simulink model "V4_Event_ind_eso_auxi"  (R2021b)
settings: Solver=ode5  StartTime=0.0  StopTime=60.0  FixedStep=0.008  RelTol=1e-3
settings Model: Creator=a1752760  LastModifiedBy=MikeYang

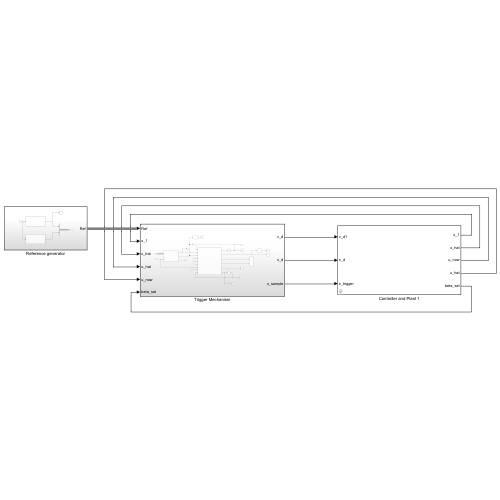
[thumbnail: Simulink's stored preview of the top-level diagram]
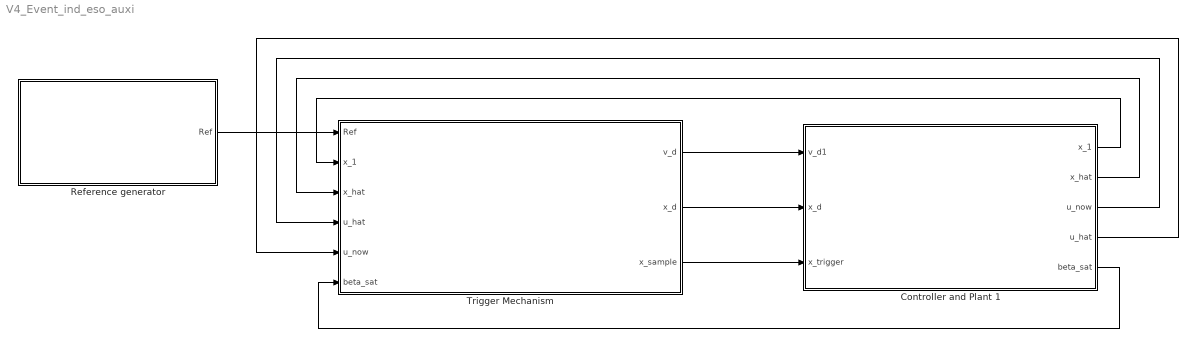
== system V4_Event_ind_eso_auxi ==
  Controller and Plant 1 : Subsystem  mask{InitialCondition=[0.8;-1.1;pi/50], UpperLimit=0.2, LowerLimit=-0.2}
      mask prompts: InitialCondition "Simulink:blkprm_prompts:IntegratorInitCond"; UpperLimit "Simulink:blkprm_prompts:SaturateUpLim"; LowerLimit "Simulink:blkprm_prompts:SaturateLowLim"
      mask TypeOptions InitialCondition: x_int/InitialCondition
      mask TypeOptions UpperLimit: Saturation/UpperLimit
      mask TypeOptions LowerLimit: Saturation/LowerLimit
      mask DialogControl InitialCondition Prompt: 初始条件:
      mask DialogControl UpperLimit Prompt: 上限:
      mask DialogControl LowerLimit Prompt: 下限:
  Reference generator : Subsystem
  Trigger Mechanism : Subsystem
  wires:
  Reference generator/1(Ref) -> Trigger Mechanism/1(Ref)
  Trigger Mechanism/1(v_d) -> Controller and Plant 1/1(v_d1)
  Trigger Mechanism/2(x_d) -> Controller and Plant 1/2(x_d)
  Controller and Plant 1/1(x_1) -> Trigger Mechanism/2(x_1)
  Trigger Mechanism/3(x_sample) -> Controller and Plant 1/3(x_trigger)
  Controller and Plant 1/2(x_hat) -> Trigger Mechanism/3(x_hat)
  Controller and Plant 1/3(u_now) -> Trigger Mechanism/4(u_hat)
  Controller and Plant 1/4(u_hat) -> Trigger Mechanism/5(u_now)
  Controller and Plant 1/5(beta_sat) -> Trigger Mechanism/6(beta_sat)

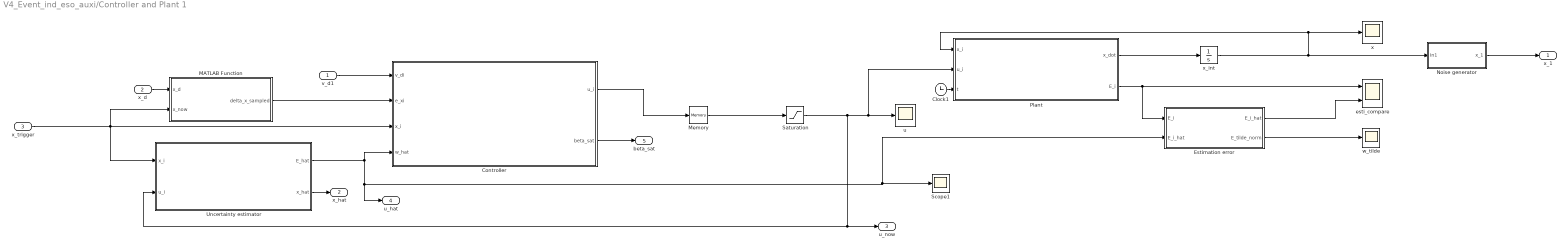
== system V4_Event_ind_eso_auxi/Controller and Plant 1 ==
  v_d1 : Inport
  x_d : Inport  Port=2
  x_trigger : Inport  Port=3
  Clock1 : Clock
  Controller : Subsystem
  Estimation error : MATLAB Function  TreatAsAtomicUnit=on
  MATLAB Function : MATLAB Function  TreatAsAtomicUnit=on
  Memory : Memory  InitialCondition=[0;0;0]
  Noise generator : Subsystem
  Plant : MATLAB Function  TreatAsAtomicUnit=on
  Saturation : Saturate  UpperLimit=UpperLimit  LowerLimit=LowerLimit
  Scope1 : Scope
  Uncertainty estimator : Subsystem  mask{x_hat_1=[0.8;-1.1;pi/50]}
      mask prompts: x_hat_1 "Simulink:blkprm_prompts:IntegratorInitCond"
      mask TypeOptions x_hat_1: Integrator/InitialCondition
      mask DialogControl x_hat_1 Prompt: 初始条件:
  esti_compare : Scope  NumInputPorts=2
  u : Scope
  w_tilde : Scope
  x : Scope
  x_int : Integrator  InitialCondition=InitialCondition
  x_1 : Outport
  x_hat : Outport  Port=2
  u_now : Outport  Port=3
  u_hat : Outport  Port=4
  beta_sat : Outport  Port=5
  wires:
  Plant/2(E_i) -> esti_compare/1, Estimation error/1(E_i)
  Uncertainty estimator/1(E_hat) -> Controller/4(w_hat), u_hat/1, Estimation error/2("E_i_hat "), Scope1/1
  Clock1/1 -> Plant/3(t)
  Plant/1(x_dot) -> x_int/1
  Memory/1 -> Saturation/1
  x_int/1 -> Noise generator/1(In1), Plant/1(x_i), x/1
  v_d1/1 -> Controller/1(v_di)
  Controller/1(u_i) -> Memory/1
  Saturation/1 -> u_now/1, Uncertainty estimator/2(u_i), Plant/2(u_i), u/1
  Estimation error/2(E_tilde_norm) -> w_tilde/1
  Estimation error/1(E_i_hat) -> esti_compare/2
  MATLAB Function/1(delta_x_sampled) -> Controller/2(e_xi)
  x_trigger/1 -> Uncertainty estimator/1(x_i), MATLAB Function/2(x_now), Controller/3(x_i)
  x_d/1 -> MATLAB Function/1(x_d)
  Uncertainty estimator/2(x_hat) -> x_hat/1
  Noise generator/1(x_1) -> x_1/1
  Controller/2(beta_sat) -> beta_sat/1

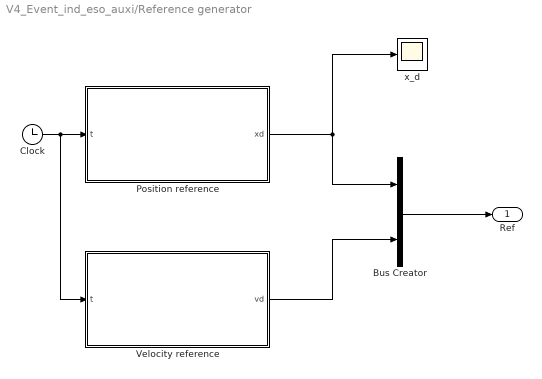
== system V4_Event_ind_eso_auxi/Reference generator ==
  Bus Creator : BusCreator  Inputs=2
  Clock : Clock
  Position reference : MATLAB Function  TreatAsAtomicUnit=on
  Velocity reference : MATLAB Function  TreatAsAtomicUnit=on
  x_d : Scope
  Ref : Outport
  wires:
  Clock/1 -> Velocity reference/1(t), Position reference/1(t)
  Position reference/1(xd) -> x_d/1, Bus Creator/1
  Velocity reference/1(vd) -> Bus Creator/2
  Bus Creator/1 -> Ref/1

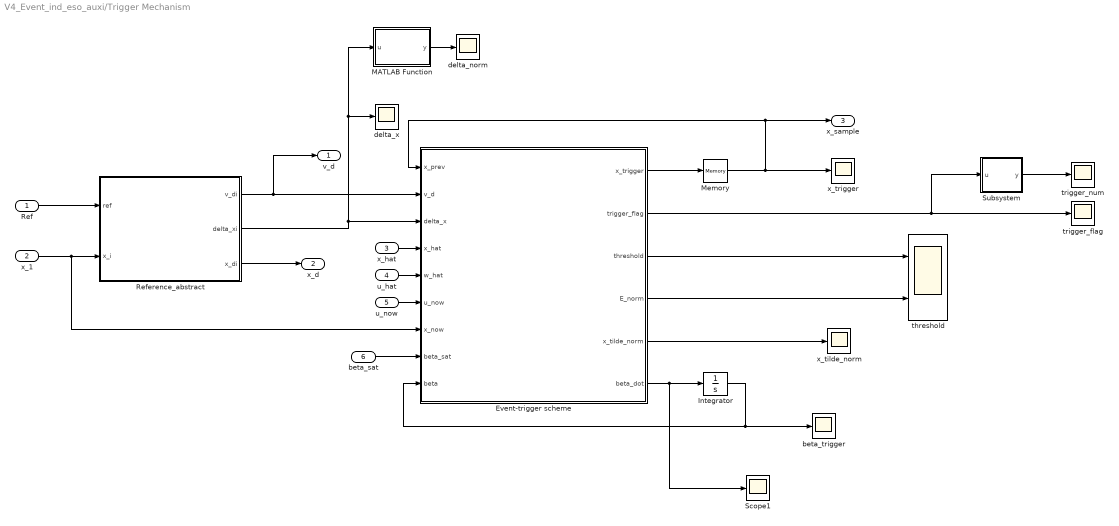
== system V4_Event_ind_eso_auxi/Trigger Mechanism ==
  Ref : Inport
  x_1 : Inport  Port=2
  x_hat : Inport  Port=3
  u_hat : Inport  Port=4
  u_now : Inport  Port=5
  beta_sat : Inport  Port=6
  Event-trigger scheme : MATLAB Function  TreatAsAtomicUnit=on
  Integrator : Integrator  InitialCondition=[2;2]
  MATLAB Function : MATLAB Function  TreatAsAtomicUnit=on
  Memory : Memory  InitialCondition=[0.8;-1.1;pi/50]
  Reference_abstract : MATLAB Function  TreatAsAtomicUnit=on
  Scope1 : Scope
  Subsystem : Subsystem
  beta_trigger : Scope
  delta_norm : Scope
  delta_x : Scope
  threshold : Scope  NumInputPorts=2
  trigger_flag : Scope
  trigger_num : Scope
  x_tilde_norm : Scope
  x_trigger : Scope
  v_d : Outport
  x_d : Outport  Port=2
  x_sample : Outport  Port=3
  wires:
  Ref/1 -> Reference_abstract/1(ref)
  Reference_abstract/1(v_di) -> Event-trigger scheme/2(v_d), v_d/1
  x_1/1 -> Event-trigger scheme/7(x_now), Reference_abstract/2(x_i)
  Event-trigger scheme/1(x_trigger) -> Memory/1
  Memory/1 -> x_trigger/1, x_sample/1, Event-trigger scheme/1(x_prev)
  Reference_abstract/2(delta_xi) -> MATLAB Function/1(u), delta_x/1, Event-trigger scheme/3(delta_x)
  Reference_abstract/3(x_di) -> x_d/1
  x_hat/1 -> Event-trigger scheme/4(x_hat)
  u_hat/1 -> Event-trigger scheme/5(w_hat)
  u_now/1 -> Event-trigger scheme/6(u_now)
  Event-trigger scheme/3(threshold) -> threshold/1
  Event-trigger scheme/4(E_norm) -> threshold/2
  Subsystem/1(y) -> trigger_num/1
  Event-trigger scheme/2(trigger_flag) -> Subsystem/1(u), trigger_flag/1
  Event-trigger scheme/5(x_tilde_norm) -> x_tilde_norm/1
  MATLAB Function/1(y) -> delta_norm/1
  Event-trigger scheme/6(beta_dot) -> Integrator/1, Scope1/1
  Integrator/1 -> beta_trigger/1, Event-trigger scheme/9(beta)
  beta_sat/1 -> Event-trigger scheme/8(beta_sat)

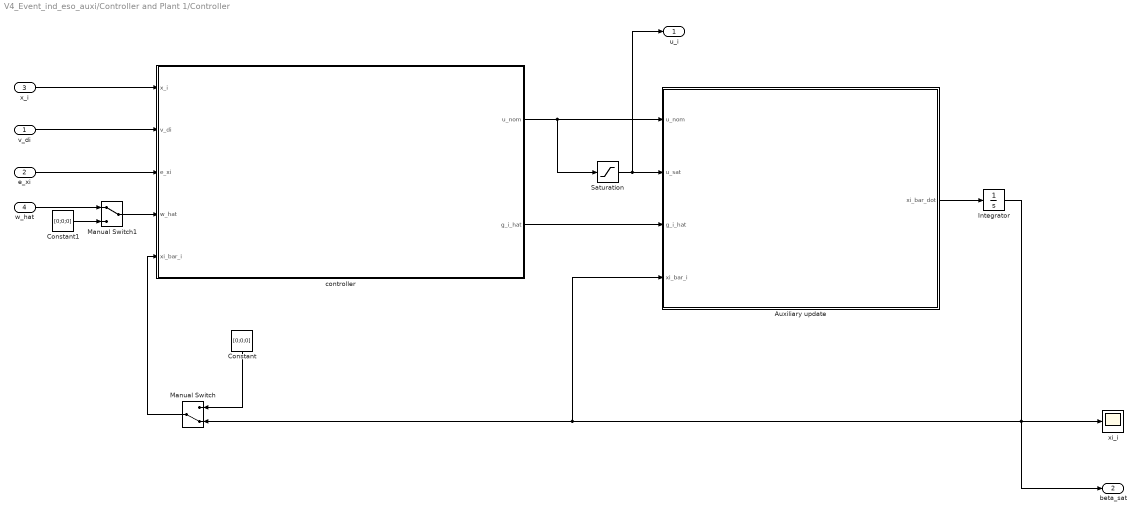
== system V4_Event_ind_eso_auxi/Controller and Plant 1/Controller ==
  v_di : Inport
  e_xi : Inport  Port=2
  x_i : Inport  Port=3
  w_hat : Inport  Port=4
  Auxiliary update : MATLAB Function  TreatAsAtomicUnit=on
  Constant : Constant  Value=[0;0;0]
  Constant1 : Constant  Value=[0;0;0]  VectorParams1D=off
  Integrator : Integrator  InitialCondition=[0.1;0.1;0.1]
  Manual Switch : ManualSwitch  CurrentSetting=0
  Manual Switch1 : ManualSwitch
  Saturation : Saturate  UpperLimit=0.2  LowerLimit=-0.2
  controller : MATLAB Function  TreatAsAtomicUnit=on
  xi_i : Scope
  u_i : Outport
  beta_sat : Outport  Port=2
  wires:
  x_i/1 -> controller/1(x_i)
  v_di/1 -> controller/2(v_di)
  e_xi/1 -> controller/3(e_xi)
  controller/1(u_nom) -> Saturation/1, Auxiliary update/1(u_nom)
  Saturation/1 -> u_i/1, Auxiliary update/2(u_sat)
  controller/2(g_i_hat) -> Auxiliary update/3(g_i_hat)
  Auxiliary update/1(xi_bar_dot) -> Integrator/1
  Constant/1 -> Manual Switch/1
  Manual Switch/1 -> controller/5(xi_bar_i)
  Integrator/1 -> beta_sat/1, xi_i/1, Auxiliary update/4(xi_bar_i), Manual Switch/2
  Constant1/1 -> Manual Switch1/2
  Manual Switch1/1 -> controller/4(w_hat)
  w_hat/1 -> Manual Switch1/1

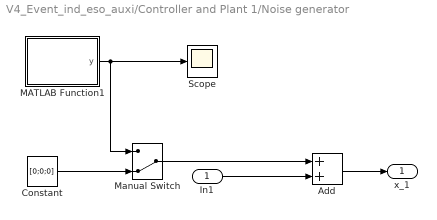
== system V4_Event_ind_eso_auxi/Controller and Plant 1/Noise generator ==
  In1 : Inport
  Add : Sum
  Constant : Constant  Value=[0;0;0]
  MATLAB Function1 : MATLAB Function  TreatAsAtomicUnit=on
  Manual Switch : ManualSwitch  CurrentSetting=0
  Scope : Scope
  x_1 : Outport
  wires:
  MATLAB Function1/1(y) -> Manual Switch/1, Scope/1
  In1/1 -> Add/2
  Add/1 -> x_1/1
  Manual Switch/1 -> Add/1
  Constant/1 -> Manual Switch/2

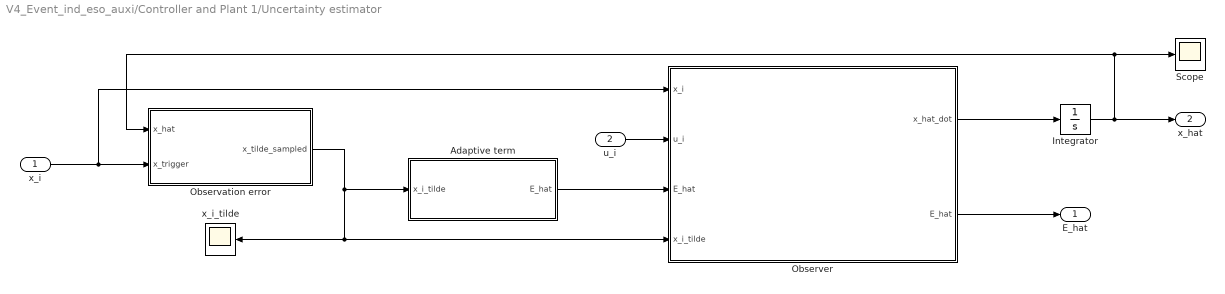
== system V4_Event_ind_eso_auxi/Controller and Plant 1/Uncertainty estimator ==
  x_i : Inport
  u_i : Inport  Port=2
  Adaptive term : Subsystem
  Integrator : Integrator  InitialCondition=x_hat_1
  Observation error : MATLAB Function  TreatAsAtomicUnit=on
  Observer : MATLAB Function  TreatAsAtomicUnit=on
  Scope : Scope
  x_i_tilde : Scope
  E_hat : Outport
  x_hat : Outport  Port=2
  wires:
  Adaptive term/1(E_hat) -> Observer/3("E_hat ")
  Observer/1(x_hat_dot) -> Integrator/1
  u_i/1 -> Observer/2(u_i)
  Integrator/1 -> Observation error/1(x_hat), Scope/1, x_hat/1
  x_i/1 -> Observation error/2(x_trigger), Observer/1(x_i)
  Observer/2(E_hat) -> E_hat/1
  Observation error/1(x_tilde_sampled) -> Observer/4(x_i_tilde), x_i_tilde/1, Adaptive term/1(x_i_tilde)

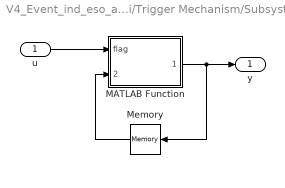
== system V4_Event_ind_eso_auxi/Trigger Mechanism/Subsystem ==
  u : Inport
  MATLAB Function : MATLAB Function  TreatAsAtomicUnit=on
  Memory : Memory
  y : Outport
  wires:
  u/1 -> MATLAB Function/1(flag)
  MATLAB Function/1(number) -> Memory/1, y/1
  Memory/1 -> MATLAB Function/2("number ")

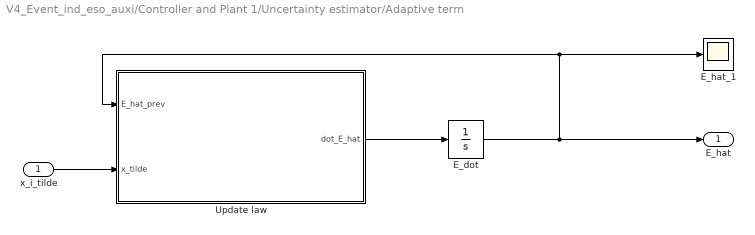
== system V4_Event_ind_eso_auxi/Controller and Plant 1/Uncertainty estimator/Adaptive term ==
  x_i_tilde : Inport
  E_dot : Integrator  InitialCondition=[0;0;0]
  E_hat_1 : Scope
  Update law : MATLAB Function  TreatAsAtomicUnit=on
  E_hat : Outport
  wires:
  E_dot/1 -> Update law/1(E_hat_prev), E_hat_1/1, E_hat/1
  x_i_tilde/1 -> Update law/2(x_tilde)
  Update law/1(dot_E_hat) -> E_dot/1

== matlab function V4_Event_ind_eso_auxi/Trigger Mechanism/Event-trigger scheme ==
  data: x_prev input; v_d input; x_trigger output; delta_x input; x_hat input; w_hat input; u_now input; x_now input; beta_sat input; trigger_flag output; threshold output; E_norm output; x_tilde_norm output; beta input; beta_dot output
function [x_trigger, trigger_flag, threshold, E_norm, x_tilde_norm, beta_dot] = event_trigger(x_prev, v_d, delta_x, x_hat, w_hat, u_now, x_now, beta_sat, beta)

% Observer
eta_1 = [21,21,3];
k_1 = [3,3,1];
rho_2 = 0.08;
xi_2 = 0.5;
gamma_2 = 0.6;
alpha_2 = 1;

% Controller
k_2 = [3,3,1.5];
k_3 = [8,8,2];
rho_3 = 0.08;
xi_3 = 0.5;
gamma_3 = 0.6;
alpha_3 = 1;
rho_4 = 0.08;
L_1 = 1.74;
L_2 = 1.42;

% Necessary variable
x_tilde = x_now - x_hat;
x_tilde_norm = norm(x_tilde(1:3));

% Measurement error
E_x = x_now - x_prev;

% Threshold related function
K_3 = diag(eta_1) * diag(k_1) - 2 * eye(3);
F_2 = (L_1 * norm(diag(eta_1) * u_now)^2 * norm(E_x)^2/4 + norm(diag(eta_1)* diag(k_1) * E_x)^2/4 + norm(diag(eta_1) * E_x)^2) - rho_2 * x_tilde' * K_3 * x_tilde;

% F_2 = (L_2 * norm(v_d - w_hat - diag(k_3) * beta_sat)^2 * norm(E_x)^2 + norm(diag(k_2) * E_x)^2) - rho_2 * delta_x' * (diag(k_2) - eye(3)) * delta_x;
F_3 = (L_2 * norm(v_d - w_hat - diag(k_3) * beta_sat)^2 * norm(E_x)^2 + norm(diag(k_2) * E_x)^2) - rho_3 * delta_x' * diag(k_2) * delta_x;
F_4 = max(k_2) * L_2 * norm(E_x) * norm(delta_x)^2 - rho_4 * (1 - rho_3) * (delta_x' * diag(k_2) * delta_x);
% F_3 = max(k_2) * L_2 * norm(E_x) * norm(delta_x)^2 - rho_3 * (1 - rho_2) * (delta_x' * (diag(k_2) - eye(3)) * delta_x);

beta_est = beta(1);
beta_con = beta(2);

threshold = [F_2 - gamma_2 * beta_est, F_3 - gamma_3 * beta_con, F_4];

if max(threshold) >= 0
    trigger_flag = 1;
    x_trigger = x_now;
    E_x = 0;
    F_2 = (L_1 * norm(diag(eta_1) * u_now)^2 * norm(E_x)^2/4 + norm(diag(eta_1)* diag(k_1) * E_x)^2/4 + norm(diag(eta_1) * E_x)^2) - rho_2 * x_tilde' * K_3 * x_tilde;
    F_3 = (L_2 * norm(v_d - w_hat - diag(k_3) * beta_sat)^2 * norm(E_x)^2 + norm(diag(k_2) * E_x)^2) - rho_3 * delta_x' * diag(k_2) * delta_x;
    E_norm = 0;
else
    trigger_flag = 0;
    x_trigger = x_prev;
    E_norm = norm(E_x);
end

beta_ob_dot = - alpha_2 * beta_est - F_2 + xi_2;
beta_con_dot = - alpha_3 * beta_con - F_3 + xi_3;

beta_dot = [beta_ob_dot;beta_con_dot];

% trigger_flag = 1;
% x_trigger = x_now;
% E_norm = 0;

end

== matlab function V4_Event_ind_eso_auxi/Controller and Plant 1/Uncertainty estimator/Observer ==
  data: x_i input; u_i input; x_hat_dot output; E_hat output; E_hat input; x_i_tilde input
function [x_hat_dot, E_hat] = observer(x_i, u_i, E_hat, x_i_tilde)

%% observer itself
Radius_esti=[0.13,0.13,0.13];

serial_num = 1;
dimension = 3; 

k_1 = diag([3,3,1]);
% k_1 = diag([2.5,2.5,0.5]);
% k_2 = diag([0.5,0.5,0.3]);
% p = 11/13;

R_hat=Radius_esti(serial_num);

theta = x_i(dimension);

g_i_hat = [-sin(theta) -sin(pi/3 - theta) sin(pi/3 + theta);
            cos(theta) -cos(pi/3 - theta) -cos(pi/3+ theta);
            1/R_hat 1/R_hat 1/R_hat];

u_i_hat = E_hat + k_1 * x_i_tilde;

x_hat_dot = g_i_hat * u_i + u_i_hat;

end

== matlab function V4_Event_ind_eso_auxi/Controller and Plant 1/Controller/controller ==
  data: x_i input; v_di input; u_nom output; e_xi input; w_hat input; xi_bar_i input; g_i_hat output
function [u_nom, g_i_hat] = controller(x_i, v_di, e_xi, w_hat, xi_bar_i)

%% Reverse of the control gain matrix
Radius_esti=[0.13,0.13,0.13];

serial_num = 1;
dimension = 3; 

R_hat=Radius_esti(serial_num);

theta = x_i(dimension);

g_i_hat = [-sin(theta) -sin(pi/3 - theta) sin(pi/3 + theta);
        cos(theta) -cos(pi/3 - theta) -cos(pi/3+ theta);
        1/R_hat 1/R_hat 1/R_hat];

g_inverse = g_i_hat^(-1); 

%% Nominal control input
k_2 = diag([3,3,1.5]);
k_3 = diag([8,8,2]);

u_nom = g_inverse * (- k_2 * e_xi - k_3 * xi_bar_i - w_hat + v_di);

end

== matlab function V4_Event_ind_eso_auxi/Reference generator/Position reference ==
  data: t input; xd output
function xd = x_d(t)

% bias_x=0.2*t;
% bias_y=sin(0.3*t);

bias_x= 0;
bias_y= - t/60 - 1;

radius=0.35;
w= - pi/13;

phase=0;

x1=[radius*cos(w*t+2*pi/3*1+phase)+bias_x ; 1.5 * radius*sin(w*t+2*pi/3*1+phase)+bias_y ; 0];
% x2=[radius*cos(w*t+2*pi/3*2+phase)+bias_x ; 1.5 * radius*sin(w*t+2*pi/3*2+phase)+bias_y ; 0];
% x3=[radius*cos(w*t+2*pi/3*3+phase)+bias_x ; 1.5 * radius*sin(w*t+2*pi/3*3+phase)+bias_y ; 0];

% xd=[x1;x2;x3];
xd  = x1;

end

== matlab function V4_Event_ind_eso_auxi/Reference generator/Velocity reference ==
  data: t input; vd output
function vd = v_d(t)

bias_x_v = 0;
bias_y_v = - 1/60;

radius = 0.35;
w = - pi/13;

phase = 0;

v1 = [- radius * w * sin(w*t+2*pi/3*1+phase)+bias_x_v; 1.5 * radius * w * cos(w*t+2*pi/3*1+phase) + bias_y_v; 0];
% v2=[- radius * w * sin(w*t+2*pi/3*2+phase)+bias_x_v; 1.5 * radius * w * cos(w*t+2*pi/3*2+phase) + bias_y_v; 0];
% v3=[- radius * w * sin(w*t+2*pi/3*3+phase)+bias_x_v; 1.5 * radius * w * cos(w*t+2*pi/3*3+phase) + bias_y_v; 0];

vd=v1;

end

== matlab function V4_Event_ind_eso_auxi/Controller and Plant 1/Controller/Auxiliary update ==
  data: u_nom input; xi_bar_dot output; u_sat input; g_i_hat input; xi_bar_i input
function xi_bar_dot = auxi_updata(u_nom, u_sat, g_i_hat, xi_bar_i)

eta_3 = diag([6,6,1]);

u_diff = u_nom - u_sat;

eta_4 = diag([0.5,0.5,0.2]);

if norm(xi_bar_i)>=0.005
    xi_bar_dot = eta_3 * g_i_hat * u_diff - eta_4 * xi_bar_i - 1 * norm(u_diff)^2/norm(xi_bar_i)^2 * xi_bar_i;
else
    xi_bar_dot = eta_3 * g_i_hat * u_diff - eta_4 * xi_bar_i;
end


end

== matlab function V4_Event_ind_eso_auxi/Controller and Plant 1/Plant ==
  data: x_dot output; E_i output; x_i input; u_i input; t input
function [x_dot, E_i ] = model(x_i, u_i, t)

%% First-order plants for robots
Radius=[0.13,0.13,0.13];
Radius_esti=[0.13,0.13,0.13];

serial_num = 1;

R = Radius(serial_num);
R_hat = Radius_esti(serial_num);

x = x_i(1);
y = x_i(2);
theta = x_i(3);

w_i =  [0.1 * cos(0.8* t - serial_num * pi/2); 0.1 * sin(0.8*t + serial_num * pi/3); 0.08*sin(0.1*t + serial_num * 5 *pi/4)];
%d =  0.4* cos(0.5* t+ pi/2);


g_i = [-sin(theta) -sin(pi/3 - theta) sin(pi/3 + theta);
        cos(theta) -cos(pi/3 - theta) -cos(pi/3+ theta);
        1/R 1/R 1/R];
    
g_i_hat = [-sin(theta) -sin(pi/3 - theta) sin(pi/3 + theta);
        cos(theta) -cos(pi/3 - theta) -cos(pi/3+ theta);
        1/R_hat 1/R_hat 1/R_hat];
    
x_dot = g_i * u_i + w_i;


E_i = w_i + (g_i - g_i_hat) * u_i;




end

== matlab function V4_Event_ind_eso_auxi/Trigger Mechanism/Reference_abstract ==
  data: v_di output; ref input; x_i input; delta_xi output; x_di output
function [v_di, delta_xi, x_di] = ref_obtain(ref, x_i)

%% Basic parameters

dimension = 3;
num_agent = 1;
serial_num = 1;

x_d = ref(1+dimension*0:dimension*num_agent);
v_d = ref(1+dimension*num_agent:2*dimension*num_agent);

x_di = x_d( (serial_num - 1)*dimension+1 : serial_num*dimension );
v_di = v_d( (serial_num - 1)*dimension+1 : serial_num*dimension );

delta_xi = x_i - x_di; 

end

== matlab function V4_Event_ind_eso_auxi/Controller and Plant 1/Uncertainty estimator/Observation error ==
  data: x_hat input; x_trigger input; x_tilde_sampled output
function x_tilde_sampled = error_calculation(x_hat, x_trigger)

x_tilde_sampled = x_trigger - x_hat;

end

== matlab function V4_Event_ind_eso_auxi/Controller and Plant 1/MATLAB Function ==
  data: x_d input; x_now input; delta_x_sampled output
function delta_x_sampled = tracking_error(x_d, x_now)

delta_x_sampled = x_now - x_d;

end

== matlab function V4_Event_ind_eso_auxi/Controller and Plant 1/Uncertainty estimator/Adaptive term/Update law ==
  data: E_hat_prev input; x_tilde input; dot_E_hat output
function dot_E_hat = adaptive_law(E_hat_prev, x_tilde)

eta_1 = diag([21,21,3]);
% eta_1 = diag([5,5,1.5]);
% eta_3 = diag([3,3,0.5]);
% p = 7/11;

eta_2 = 0.7;

% dot_E_hat = eta_1 * x_tilde + eta_3 * diag(sign(x_tilde)) * abs(x_tilde).^p - eta_2 * E_hat_prev;
% dot_E_hat = eta_1 * x_tilde - eta_2 * E_hat_prev;
dot_E_hat = eta_1 * x_tilde;

end

== matlab function V4_Event_ind_eso_auxi/Controller and Plant 1/Estimation error ==
  data: E_i input; E_i_hat output; E_i_hat input; E_tilde_norm output
function [E_i_hat, E_tilde_norm] = esti_error(E_i, E_i_hat)

E_i_tilde = E_i - E_i_hat;
E_tilde_norm = norm(E_i_tilde);

end

== matlab function V4_Event_ind_eso_auxi/Trigger Mechanism/MATLAB Function ==
  data: u input; y output
function y = fcn(u)

y = norm(u);

end

== matlab function V4_Event_ind_eso_auxi/Controller and Plant 1/Noise generator/MATLAB Function1 ==
  data: y output
function y = fcn()

y = diag([0.001, 0.001, 0.01]) * randn(3,1);

end

== matlab function V4_Event_ind_eso_auxi/Trigger Mechanism/Subsystem/MATLAB Function ==
  data: flag input; number output; number input
function number = counter(flag, number)

if flag == 1
    number = number + 1;
end

end
